simulink library "VisualAqSurveillanceBlock_devAlt"  (R2019b)
settings: Solver=VariableStepAuto  StartTime=0.0  StopTime=10.0  RelTol=1e-3
undefined symbols (not defined in the file): visaq_alert, visaq_area_s, visaq_beta0, visaq_beta1, visaq_d1, visaq_dlim, visaq_fovd, visaq_fovl, visaq_fovr, visaq_fovu, visaq_pl, visaq_pr, visaq_r, visaq_rseed, visaq_t1, visaq_t2, visaq_vdf, visaq_vis
libraries: CreateCovDiagMatrix x1, simulink x1
settings Model: Creator=BI28030  LastModifiedBy=ng21251
settings DataIOCC: ReturnWorkspaceOutputs=off
settings DebuggingCC: ArithmeticOperatorsInVariantConditions=warning
settings SFSimCC: CustomCodeUndefinedFunction=UseInterfaceOnly

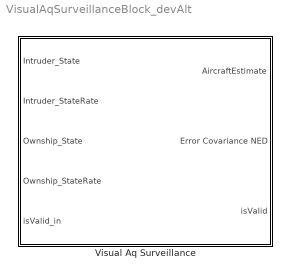
== system VisualAqSurveillanceBlock_devAlt ==
  Visual Aq Surveillance : Subsystem  Description=|  mask{dt=0.1, area_s=visaq_area_s, t2=visaq_t2, t1=visaq_t1, d1=visaq_d1, pl=visaq_pl, pr=visaq_pr, fovl=visaq_fovl, fovr=visaq_fovr, fovu=visaq_fovu, fovd=visaq_fovd, beta0=visaq_beta0, beta1=visaq_beta1, alert=visaq_alert, r=visaq_r, dlim=visaq_dlim, vis=visaq_vis, vdf=visaq_vdf, rseed=visaq_rseed}
      | Documentation for Perfect Observation Block                                                                                                                                                                                                                                                                                                                                                                                                          
      |                                                                                                                                                                                                                                                                                                                                                                                                                                                      
      | Description:  The perfect observation block, also known as a perfect                                                                                                                                                                                                                                                                                                                                                                                 
      | surveillance block, receives an Aircraft State, nominally from a Basic                                                                                                                                                                                                                                                                                                                                                                               
      | Aircraft Dynamics block, and outputs an Aircraft Estimate.  The Aircraft                                                                                                                                                                                                                                                                                                                                                                             
      | State that is received as input consists of Latitude, Longitude, and                                                                                                                                                                                                                                                                                                                                                                                 
      | Altitude state information as well as the aircraft position in local                                                                                                                                                                                                                                                                                                                                                                                 
      | coordinates in units of feet for north, east, and height.  The Aircraft                                                                                                                                                                                                                                                                                                                                                                              
      | Estimate outputs consist of estimates for the aircraft Latitude, Longitude, and Altitude, the east, north up position, and sensor covariance.  For perfect surveillance, the covariance estimates are all set to zero as default.  In addition, "time of validity" and a Boolean flag for the sensor report, "is Valid", are outputted as part of the Aircraft Estimate.                                                                             
      |                                                                                                                                                                                                                                                                                                                                                                                                                                                      
      | The initial perfect surveillance block developed receives the aircraft state information from the "AC2 - Basic Aircraft Dynamics" block within the "nominalEncounter" study.  Since the expected output from the AC1 and AC2 aircraft states have slightly different output parameters than what is provided from the perfect surveillance block (i.e., covariance estimates, isValid, and time of validity), the perfect surveillance block         
      | AircraftEstimate output has been left disconnected.                                                                                                                                                                                                                                                                                                                                                                                                  
      |                                                                                                                                                                                                                                                                                                                                                                                                                                                      
      | The initial unit test performed for this perfect observation block was to                                                                                                                                                                                                                                                                                                                                                                            
      | run the nominalEncounter study and to ensure that the simulation completes and no exceptions are encountered.  This unit test was successful (other than receiving a warning that the output of the perfect surveillance block is not connected, which was expected).  A more comprehensive future unit test would be to evaluate the position inputs and compare them with the position outputs to ensure that they are consistent with one another.
      mask prompts: dt "Dynamics Update Step Size (s)"; area_s "Aircraft Surface Area Array"; t2 "Evaluation Period (seconds)"; t1 "Alert Evaluation Period (seconds)"; d1 "Alert Evaluation Distance (nm)"; pl "Left Pilot Search Rate (0-1)"; pr "Right Pilot Search Rate (0-1)"; fovl "Pilot FOV Left (degrees ex:-110)"; fovr "Pilot FOV Right (degrees ex: 90)"; fovu "Pilot FOV Up (degrees ex:30)"; fovd "Pilot FOV Down (degrees ex: -20)"; beta0 "Beta for unalerted search (17000)"; beta1 "Beta for alerted search (14000)"; alert "Use Alerting Flag (1=yes, 0=no)"; r "R visual range (nm)"; dlim "Resolution limit of eye (arc-min)"; vis "visbility factor (0-1)"; vdf "visual degredation factor (0-1)"; rseed "Random seed for uniform distribution (0-1)"

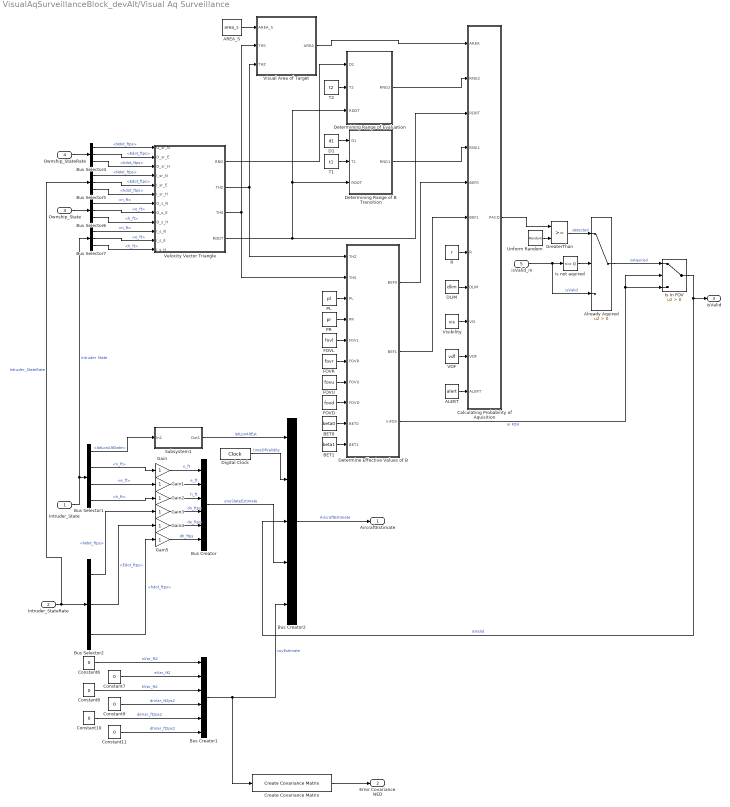
== system VisualAqSurveillanceBlock_devAlt/Visual Aq Surveillance ==
  Intruder_State : Inport  OutDataTypeStr=Bus: AircraftState
  Intruder_StateRate : Inport  Port=2  OutDataTypeStr=Bus: AircraftStateRate
  Ownship_State : Inport  Port=3  OutDataTypeStr=Bus: AircraftState
  Ownship_StateRate : Inport  Port=4  OutDataTypeStr=Bus: AircraftStateRate
  isValid_in : Inport  Port=5
  ALERT : Constant  Value=alert
  "AREA_S " : Constant  Value=area_s  VectorParams1D=off
  Already Aquired : Switch  Criteria=u2 > Threshold
  BET0 : Constant  Value=beta0
  BET1 : Constant  Value=beta1
  Bus Creator : BusCreator  Inputs=6  OutDataTypeStr=Bus: StateEstimate
  Bus Creator1 : BusCreator  Inputs=6  OutDataTypeStr=Bus: CovarianceEstimate
  Bus Creator2 : BusCreator  Inputs=5  OutDataTypeStr=Bus: AircraftEstimate  NonVirtualBus=on
  Bus Selector1 : BusSelector  OutputSignals=latLonAltState,n_ft,e_ft,h_ft
  Bus Selector2 : BusSelector  OutputSignals=Ndot_ftps,Edot_ftps,hdot_ftps
  Bus Selector4 : BusSelector  OutputSignals=Ndot_ftps,Edot_ftps,hdot_ftps
  Bus Selector5 : BusSelector  OutputSignals=Ndot_ftps,Edot_ftps,hdot_ftps
  Bus Selector6 : BusSelector  OutputSignals=n_ft,e_ft,h_ft
  Bus Selector7 : BusSelector  OutputSignals=n_ft,e_ft,h_ft
  Calculating Probability of Aquisition : MATLAB Function  TreatAsAtomicUnit=on
  Constant{6..11} (6 alike) : Constant  Value=0
  Create Covariance Matrix : CreateCovDiagMatrix/Create Covariance Matrix  SystemSampleTime=-1  Latency=0  AutoFrameSizeCalculation=off
  D1 : Constant  Value=d1
  DLIM : Constant  Value=dlim
  Determine Effective Values of B : MATLAB Function  TreatAsAtomicUnit=on
  Determining Range of B Transition : MATLAB Function  TreatAsAtomicUnit=on
  Determining Range of Evaluation : MATLAB Function  TreatAsAtomicUnit=on
  Digital Clock : DigitalClock  SampleTime=dt
  FOVD : Constant  Value=fovd
  FOVL : Constant  Value=fovl
  FOVR : Constant  Value=fovr
  FOVU : Constant  Value=fovu
  Gain{,1..5} (6 alike) : Gain
  GreaterThan : RelationalOperator  OutDataTypeStr=boolean  RndMeth=Simplest
  Is In FOV : Switch  Criteria=u2 > Threshold
  PL : Constant  Value=pl
  PR : Constant  Value=pr
  R : Constant  Value=r
  Subsystem1 : Subsystem
  T1 : Constant  Value=t1
  T2 : Constant  Value=t2
  Unform Random : UniformRandomNumber  Minimum=0  Seed=rseed  SampleTime=0.1
  VDF : Constant  Value=vdf
  Velocity Vector Triangle : MATLAB Function  TreatAsAtomicUnit=on
  Visibility : Constant  Value=vis
  Visual Area of Target : MATLAB Function  TreatAsAtomicUnit=on
  is not aquired : simulink/Logic and Bit Operations/Compare To Zero  relop=<=  OutDataTypeStr=boolean
  AircraftEstimate : Outport  OutDataTypeStr=Bus: AircraftEstimate  VectorParamsAs1DForOutWhenUnconnected=off
  Error Covariance NED : Outport  Port=2  VectorParamsAs1DForOutWhenUnconnected=off
  "isValid " : Outport  Port=3
  wires:
  Gain5/1 -> Bus Creator/6  "dh_ftps"
  Gain4/1 -> Bus Creator/5  "de_ftps"
  Gain3/1 -> Bus Creator/4  "dn_ftps"
  Gain2/1 -> Bus Creator/3  "h_ft"
  Gain1/1 -> Bus Creator/2  "e_ft"
  Gain/1 -> Bus Creator/1  "n_ft"
  Subsystem1/1(Out1) -> Bus Creator2/1  "latLonAltEst"
  Digital Clock/1 -> Bus Creator2/2  "timeOfValidity"
  isValid_in/1 -> is not aquired/1, Already Aquired/3  "isValid"
  Bus Selector1/1 -> Subsystem1/1(In1)  "<latLonAltState>"
  Bus Selector2/3 -> Gain5/1  "<hdot_ftps>"
  Bus Selector2/2 -> Gain4/1  "<Edot_ftps>"
  Bus Selector2/1 -> Gain3/1  "<Ndot_ftps>"
  Bus Selector1/4 -> Gain2/1  "<h_ft>"
  Bus Selector1/3 -> Gain1/1  "<e_ft>"
  Bus Selector1/2 -> Gain/1  "<n_ft>"
  Constant11/1 -> Bus Creator1/6  "dhVar_ft2ps2"
  Constant10/1 -> Bus Creator1/5  "deVar_ft2ps2"
  Constant9/1 -> Bus Creator1/4  "dnVar_ft2ps2"
  Constant8/1 -> Bus Creator1/3  "hVar_ft2"
  Constant7/1 -> Bus Creator1/2  "eVar_ft2"
  Constant6/1 -> Bus Creator1/1  "nVar_ft2"
  Bus Creator2/1 -> AircraftEstimate/1  "AircraftEstimate"
  Bus Creator1/1 -> Create Covariance Matrix/1, Bus Creator2/5  "covEstimate"
  Bus Creator/1 -> Bus Creator2/4  "enuStateEstimate"
  Create Covariance Matrix/1 -> Error Covariance NED/1
  Intruder_State/1 -> Bus Selector7/1, Bus Selector1/1  "Intruder State"
  Intruder_StateRate/1 -> Bus Selector5/1, Bus Selector2/1  "Intruder_StateRate"
  Bus Selector4/3 -> Velocity Vector Triangle/3(O_sr_H)  "<hdot_ftps>"
  Bus Selector4/1 -> Velocity Vector Triangle/1(O_sr_N)  "<Ndot_ftps>"
  Bus Selector4/2 -> Velocity Vector Triangle/2(O_sr_E)  "<Edot_ftps>"
  Ownship_StateRate/1 -> Bus Selector4/1
  Bus Selector5/2 -> Velocity Vector Triangle/5(I_sr_E)  "<Edot_ftps>"
  Bus Selector5/3 -> Velocity Vector Triangle/6(I_sr_H)  "<hdot_ftps>"
  Bus Selector5/1 -> Velocity Vector Triangle/4(I_sr_N)  "<Ndot_ftps>"
  Ownship_State/1 -> Bus Selector6/1
  Bus Selector6/3 -> Velocity Vector Triangle/9(O_s_H)  "<h_ft>"
  Bus Selector6/1 -> Velocity Vector Triangle/7(O_s_N)  "<n_ft>"
  Bus Selector6/2 -> Velocity Vector Triangle/8(O_s_E)  "<e_ft>"
  Bus Selector7/3 -> Velocity Vector Triangle/12(I_s_H)  "<h_ft>"
  Bus Selector7/1 -> Velocity Vector Triangle/10(I_s_N)  "<n_ft>"
  Bus Selector7/2 -> Velocity Vector Triangle/11(I_s_E)  "<e_ft>"
  Velocity Vector Triangle/4(RDOT) -> Calculating Probability of Aquisition/3(RDOT), Determining Range of Evaluation/3(RDOT), Determining Range of B Transition/3(RDOT)
  Velocity Vector Triangle/3(THS) -> Determine Effective Values of B/2(THS), Visual Area of Target/2(THS)
  D1/1 -> Determining Range of B Transition/1(D1)
  T1/1 -> Determining Range of B Transition/2(T1)
  T2/1 -> Determining Range of Evaluation/2(T2)
  Velocity Vector Triangle/1(RNG) -> Determining Range of Evaluation/1(D2)
  PL/1 -> Determine Effective Values of B/3(PL)
  PR/1 -> Determine Effective Values of B/4(PR)
  FOVL/1 -> Determine Effective Values of B/5(FOVL)
  FOVR/1 -> Determine Effective Values of B/6(FOVR)
  BET0/1 -> Determine Effective Values of B/9(BET0)
  BET1/1 -> Determine Effective Values of B/10(BET1)
  Determining Range of B Transition/1(RNG1) -> Calculating Probability of Aquisition/4(RNG1)
  Visual Area of Target/1(AREA) -> Calculating Probability of Aquisition/1(AREA)
  Determining Range of Evaluation/1(RNG2) -> Calculating Probability of Aquisition/2(RNG2)
  Determine Effective Values of B/1(BEF0) -> Calculating Probability of Aquisition/5(BEF0)
  Determine Effective Values of B/2(BEF1) -> Calculating Probability of Aquisition/6(BEF1)
  DLIM/1 -> Calculating Probability of Aquisition/8(DLIM)
  R/1 -> Calculating Probability of Aquisition/7(R)
  Velocity Vector Triangle/2(THZ) -> Determine Effective Values of B/1(THZ), Visual Area of Target/3(THZ)
  FOVU/1 -> Determine Effective Values of B/7(FOVU)
  FOVD/1 -> Determine Effective Values of B/8(FOVD)
  Calculating Probability of Aquisition/1(PACQ) -> GreaterThan/1
  Unform Random/1 -> GreaterThan/2
  GreaterThan/1 -> Already Aquired/1  "detected"
  is not aquired/1 -> Already Aquired/2
  Determine Effective Values of B/3(inFOV) -> Is In FOV/3, Is In FOV/2  "in FOV"
  Already Aquired/1 -> Is In FOV/1  "isAquired"
  Is In FOV/1 -> "isValid "/1, Bus Creator2/3  "isValid"
  VDF/1 -> Calculating Probability of Aquisition/10(VDF)
  Visibility/1 -> Calculating Probability of Aquisition/9(VIS)
  "AREA_S "/1 -> Visual Area of Target/1(AREA_S)
  ALERT/1 -> Calculating Probability of Aquisition/11(ALERT)

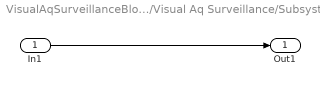
== system VisualAqSurveillanceBlock_devAlt/Visual Aq Surveillance/Subsystem1 ==
  In1 : Inport
  Out1 : Outport  VectorParamsAs1DForOutWhenUnconnected=off
  wires:
  In1/1 -> Out1/1

== matlab function VisualAqSurveillanceBlock_devAlt/Visual Aq Surveillance/Velocity Vector Triangle ==
  data: RNG output; THZ output; O_sr_N input; THS output; O_sr_E input; RDOT output; O_sr_H input; I_sr_N input; I_sr_E input; I_sr_H input; O_s_N input; O_s_E input; O_s_H input; I_s_N input; I_s_E input; I_s_H input
function [RNG, THZ, THS, RDOT] = JAndrews_Mod_2(O_sr_N,O_sr_E,O_sr_H,I_sr_N,I_sr_E,I_sr_H,O_s_N,O_s_E,O_s_H,I_s_N,I_s_E,I_s_H)
% Input variable defintions
% No, symbol, name, value, definition
% 1.  - , BET0, 17000 per steradian-sec,  single pilot B values before transition
% 2.  - , BET1, 17000 per steradian-sec,  Single-pilot B value after transition
% 3.  t1, T1,   180 sec,                  modified tau time for B transition (time to closest approach)
% 4.  t2, T2,   12 sec,                   modified tau time for evaluation of PACQ (time to closest approach)
% 5.  D1, D1,   0. nmi,                   modified tau range parameter for B transition.
% 6.  D2, D2,   0. nmi,                   modified tau range parameter for PACQ evaluation
% 7.  R,  R,    20. nmi,                  visual range
% 8.  d,  DLIM, 1 arc-min,                Resolution limit of human eye.
% 9.  V1, VSUB1,180 kt,                   airspeed of subject aircraft.
% 10. V2, VSUB2,130 kt,                   airspeed of target aircraft.
% 11. - , IACT, 1,                        aircraft type for target aircraft (see table)
% 12. X,  XANG, 180. deg,                 Crossing angle (relative heading)
% 13. PL, PL,   1.0,                      Search intensity for pilot in left seat (0 = no pilot, 1 = normal search)
% 14. PR, PR,   1.0,                      Search intensity for pilot in right seat (0 = no pilot, 1 = normal search)
% 15. FL, FOVL, -120 degrees              Field-of-view cutoff on left side for searching pilot in left seat (measured positive clockwise from straight ahead). 
% 16. FR, FOVR, -90 degrees               Field-of-view cutoff on left side for searching pilot in right seat (measured positive clockwise from straight ahead). 
% 17. r., RDOT, 380 kt*,                  Range rate of target aircraft
% 18. Ax, AX,   35 sq.ft.*,               Head-on visual area of target.
% 19. Ay, AY,   85 sq.ft.*,               Broadside visual area of target.
% 20. Az, AZ,   260 sq.ft.*,              Topside visual area of target.
% 21. A,  AREA, 35 sq.ft.*,               Final visual area of target.
% 22. 0T, TH1(THS),  0 deg*,                   Bearing of target aircraft as seen from subject aircraft.
% 23. 0S, TH2(THT),  0 deg*,                   Bearing of subject aircraft as seen from target aircraft.
% 24. R1, RNG1, 3.78 nmi*,                Range at which B transition occurs.
% 25. R2, RNG2, 1.27 nmi*,                Range at which PACQ is evaluated.
% 26. B0, BEF0, 17000* per steradian-sec, Effective value of B before transition.
% 27. B1, BEF1, 17000* per steradian-sec, Effective value of B after transition.
% 28. P, PACQ,  -                         Probability of visual aquisition
% *=value that is computed when all 16 input variables have nominal value.

%% Module 2 Description - - - - - - - 
% From a knowledge of the aircraft airspeeds and the croesing angle,
% Module 2 solves the velocity vector triangle (Fig. 4.4) to determine the
% epPrOach bearings and range rate. This solution assumes that the aircraft are
% on a rectilinear collision course and hence that the horizontal fiss distance
% is zero. For theee conditions, the valuea of the range rate (R~) and the
% approach bearings (THS and THT) are constant.

% Approach bearings are meaeured positive clockwise from straight ahead and
% are expreesed as a number between -180 degraes and +180 degreee. me crossing
% angle, NG, ie simply the relative heading formed by subtracting the headiog
% of the target aircraft from the heading of the subject aircraft. The simple
% trigonometric formula that relatee the approach bearinge and the crossing
% angle is

% WG = 180° + THS - THT

% me approach bearing for the target aircraft (THT) is important since it
% detetines the vieual area that will be seen from the subject aircraft (see
% discussion in 4.2.3). The approach bearing for the subject (~S) is usad in
% Module 4 to determine whethar or not the target ia within the cockpit
% field-of~few.

%% --------------------Module 2 ------------------
%Output
%THT - 
%THS (degrees)
%RDOT (knots)
%RNG (nm)

%get heading of Ownship (degrees)
VSUB=rad2deg(pi/2 - atan2(O_sr_N, O_sr_E));

%get heading of intruder (degrees)
VTAR=rad2deg(pi/2 - atan2(I_sr_N, I_sr_E));

%bearing to intruder (from ownship) (degrees)

    %intruder location (if ownship was at 0,0)
    Int_loc=[I_s_N - O_s_N, I_s_E - O_s_E];

    %Bearing to intruder from ownship (degrees)
    THS = rad2deg( pi/2 - atan2( Int_loc(1), Int_loc(2) ) );
    
%bearing to ownship (from intruder) (degrees)

    %ownship location (if intruder was at 0,0)
    Own_loc=[O_s_N - I_s_N, O_s_E - I_s_E];
    
    %bearing to ownship from intruder (degrees)
    THT = rad2deg( pi/2 - atan2( Own_loc(1), Own_loc(2) ) );

%check that intruder & own bearings math is correct.
% assert(isequal(ceil(sum(THT,THS)),360));

%calculate the difference between headings
XANG= 180 + THS - THT;

%Calculate RDOT - range rate
RDOT_ftsec = ( (I_sr_N - O_sr_N)^2 + (I_sr_E - O_sr_E)^2 )^(1/2);
RDOT = RDOT_ftsec * 60*60 / 6076.115486; %now in knots

%Calculate THZ in degrees

    %calculate adjacent - horizontal distance
    H_dist = ( (I_s_N - O_s_N)^2 + (I_s_E - O_s_E)^2 )^0.5;

    %calculate opposite - vertical distance
    V_dist = I_s_H - O_s_H;

    %calculate vertical angle
    THZ = rad2deg( atan(V_dist / H_dist));
    
RNG = ( (I_s_N - O_s_N)^2 + (I_s_E - O_s_E)^2 )^(1/2);

== matlab function VisualAqSurveillanceBlock_devAlt/Visual Aq Surveillance/Visual Area of Target ==
  data: AREA_S input; AREA output; THS input; THZ input
function AREA = JAndrews_Mod_3(AREA_S, THS, THZ)
% Input variable defintions
% No, symbol, name, value, definition
% 18. Ax, AX,   35 sq.ft.*,               Head-on visual area of target.
% 19. Ay, AY,   85 sq.ft.*,               Broadside visual area of target.
% 20. Az, AZ,   260 sq.ft.*,              Topside visual area of target.
% 21. A,  AREA, 35 sq.ft.*,               Final visual area of target.
% 22. 0T, TH1,  0 deg*,                   Bearing of target aircraft as seen from subject aircraft.
% 23. 0S, TH2,  0 deg*,                   Bearing of subject aircraft as seen from target aircraft.
% 24. R1, RNG1, 3.78 nmi*,                Range at which B transition occurs.
% 25. R2, RNG2, 1.27 nmi*,                Range at which PACQ is evaluated.
% 26. B0, BEF0, 17000* per steradian-sec, Effective value of B before transition.
% 27. B1, BEF1, 17000* per steradian-sec, Effective value of B after transition.
% 28. P, PACQ,  -                         Probability of visual aquisition
% *=value that is computed when all 16 input variables have nominal value.



%%-------MODULE 3---------
% 4.2.3 Module 3: Computing the Visual Area of the Target
% The visual area of the target ie computed by projecting the principal
% visual areas AX and AY onto a plane that is normal to the linemf-sfght
% between the two aircraft. ~is plane is at an angle ~ with respect to the
% Y-Z plane for the target aircraft. h approximate correction for shielding ie
% applied by assudng that the actual visual area is the largest of the
% projectione of M and AY plus one+hird of the smallest projection (see
% Mference 2). ~is approximation is errorless when the aircraft ie viewed
% along one of the principal axas. Because Mdule 3 assumes that the
% line-f =ight lies tithin the X-Y plane, the topside area, AZ, ie not allowed
% to centribute to the target visual area. This ia normally a good assumption,
% but can result in underestimation of the visual area if the pitch angle of the
% aircraft is large. U is defined in the module to allow for future exteneion
% of the software.




    
    THSdiff=abs(AREA_S(:,1)-THS);
    THZdiff=abs(AREA_S(:,2)-THZ);
    TOTdiff=THSdiff+THZdiff;
    mindiff=min(TOTdiff);
    
    %find the closest angle combination
    indx=ismember(TOTdiff,mindiff);
    
    %make a list of indicies
    %find the incidices that are the closest
    %take the first instance only
    indxnum=1:numel(indx);
    indxnum=indxnum(indx>0);
    indxnum=indxnum(1);
    
    %area = first smallest index - convert to nm^2
    AREA=AREA_S(indxnum,3)/6076.115486;
    
    
% else
% 
% XArea = abs(cos(deg2rad(THS))) * abs(cos(deg2rad(THZ))) * AX;
% YArea = abs(sin(deg2rad(THS))) * abs(cos(deg2rad(THZ))) * AY;
% 
% ZArea = abs(sin(deg2rad(THZ))) * AZ;
% 
% 
% 
% AREA = XArea + YArea + ZArea;
% AREA=AREA/6076.115486;
% end

== matlab function VisualAqSurveillanceBlock_devAlt/Visual Aq Surveillance/Determining Range of B Transition ==
  data: D1 input; RNG1 output; T1 input; RDOT input
function RNG1 = JAndrews_Mod_6(D1,T1,RDOT)
% Input variable defintions
% No, symbol, name, value, definition
% 3.  t1, T1,   180 sec,                  modified tau time for B transition (time to closest approach)
% 5.  D1, D1,   0. nmi,                   modified tau range parameter for B transition.
% 17. r., RDOT, 380 kt*,                  Range rate of target aircraft
% 24. R1, RNG1, 3.78 nmi*,                Range at which B transition occurs.
% *=value that is computed when all 16 input variables have nominal value.

%% Modeule 6 -
% 4.2.6 Wdule 6: Determining the tinge of 8 Transition
% In a particular scenario, the nominal value of 6 for a single pilot mey
% be alterad by an event such as the receipt of a traffic advieory.SEE1 allowa
% the notinal single~ilot value of 6 to transition from one value to another at
% a predefined point during the encounter. The initial value of 6 is BETO.
% After the transition, the value of B fa BET1 (see Fig. 4.6). The range at
% which trzaaition occurs ia NG1. It is computed using a modified tau
% criterion involving the two input parameter DI and RI:
% 
% RNG1 = D1 - ROOT*T1
% 
% The transition occurs when the target is T1 secondefrom reaching a
% range D1. Note that if TI=O, then a simple range criterion results. H D1=O,
% then a simple time-to-collision criterion reeulta.
% If the application of interest does not require a transition, the
% transition ie easily avoided by setting BET1 equal to BETO. The eettings of
% D1 and T1 then have no effect upon the computations (becauae the valuee of 8
% are unchanged by reaching the transition point).

%RNG1 = D1 (0 nmi) - RDOT (kts) * T1 (seconds)

RNG1 = D1 - RDOT * T1;

== matlab function VisualAqSurveillanceBlock_devAlt/Visual Aq Surveillance/Determining Range of Evaluation ==
  data: D2 input; RNG2 output; T2 input; RDOT input
function RNG2 = JAndrews_Mod_5(D2, T2, RDOT)
% Input variable defintions
% No, symbol, name, value, definition
% 4.  t2, T2,   12 sec,                   modified tau time for evaluation of PACQ (time to closest approach)
% 6.  D2, D2,   0. nmi,                   modified tau range parameter for PACQ evaluation
% 17. r., RDOT, 380 kt*,                  Range rate of target aircraft
% 25. R2, RNG2, 1.27 nmi*,                Range at which PACQ is evaluated.
% *=value that is computed when all 16 input variables have nominal value.

%%  4.2.5 Module 5: Determining the ~nge of Evaluation
% The cumulative probability of visual acquisition, PACQ, depends upon the
% range, MG2, at which PACQ ia to be evaluated: Often it ia desirable to aet
% this ranga to the latest point at which sufficient time exists for evasive
% action. Then PACQ till repreeent tha probability of visual acquisition with
% aufficient lead time for avoidanca.
% RNG2 ie computed using a modified tau criterion based upon two input
% parameter D2 and U:
% ~G2 = D2 - ~OT*T2
% From thie equation it can be seen that SNG2 ie reached when tbe target
% ia T2 seconds from reaching a range of D2. with this formulation, WG2 can
% be deterdned as either a constant range, a constant time-to-collision, or a
% modified tau criterion. For example, if T2=0, then the equation yields a
% simple range critaria for which PACQ is evaluated at range D2. If D2=0,
% then a simple time critaria results in which PACQ La evaluated when T2
% secoada remain befora collision. If neither T2 nor D2 are zero, then a
% modified tau criterion results.

%RNG2 = D2 (0 nmi) - RDOT (kts) * T2 (12 seconds)

RNG2 = D2 - RDOT * T2;

== matlab function VisualAqSurveillanceBlock_devAlt/Visual Aq Surveillance/Determine Effective Values of B ==
  data: THZ input; THS input; BEF0 output; PL input; PR input; FOVL input; FOVR input; FOVU input; FOVD input; BET0 input; BET1 input; BEF1 output; inFOV output
function [BEF0, BEF1,inFOV] = JAndrews_Mod_4(THZ, THS, PL, PR, FOVL, FOVR, FOVU, FOVD, BET0, BET1)
% Input variable defintions
% No, symbol, name, value, definition
% 1.  - , BET0, 17000 per steradian-sec,  single pilot B values before transition
% 2.  - , BET1, 17000 per steradian-sec,  Single-pilot B value after transition
% 13. PL, PL,   1.0,                      Search intensity for pilot in left seat (0 = no pilot, 1 = normal search)
% 14. PR, PR,   1.0,                      Search intensity for pilot in right seat (0 = no pilot, 1 = normal search)
% 15. FL, FOVL, -120 degrees              Field-of-view cutoff on left side for searching pilot in left seat (measured positive clockwise from straight ahead). 
% 16. FR, FOVR, 90 degrees               Field-of-view cutoff on left side for searching pilot in right seat (measured positive clockwise from straight ahead). 
% 23. 0S, TH2(THT),  0 deg*,              Bearing of subject aircraft as seen from target aircraft.
% 26. B0, BEF0, 17000* per steradian-sec, Effective value of B before transition.
% 27. B1, BEF1, 17000* per steradian-sec, Effective value of B after transition.
% 28. P, PACQ,  -                         Probability of visual aquisition
% *=value that is computed when all 16 input variables have nominal value.

%% 4.2.4 Module 4: Wtermining the Effective Values of 6
% Module 4 examinee cockpit visibility and crew complement in order to
% deterfine their effect upon search effectiveness. It does eo by taking the
% notinal single~ilot B values and ebng them to produce effective B
% values. For a single pilot devoting normal effort to visual search, the
% value of S before and afterthetransitionevent(eee4.2.6)are represented
% by parameter BETO and BET1. Module 4 computes two corresponding effective
% 8 values, BEFO and BEF1, by e-rig the 8 values for each pilot who ie able to
% contribute to visual search.
% 
% The fieldmf~iew of the cockpit is deter~ned by the variables FOW and
% FOPS (ace Fig. 4.5). It ia aesumed that the cockpit visibility ia symmetric
% and that there is no cut~ff in elevation (normally true for targeta on
% collision courses). Tfienthe target ~a outside the field-f -iew, the
% effective 6 velue is set to zero.
% By setting FL and ~, the user specifies the number of pilots that
% contribute to search for both left and right visibility limite. Normally PL
% and ~ are efther sero (no pilot in the seat) or unity (single pilot in seat
% and eearching normally). It is possible to use a value between O and 1 to
% represent a pilot who is preeent, but ia devoting less than the normal amount
% of time to visual search. Or a value greater than 1 can be used to represent
% search by an additional crew member.
% 
% For the nominal input values given in Table 3.1, it ia assumed that a
% single pilot is searching from the left seat of the aircraft (PL=l.O, pR=O.O).
% For the notinal values of croesing angle (WG-180 degrees), tha intruder is
% always within the field of view. Thus for the nominal input values, BEFO=BETO
% and BEF1=BET1.

%% CHECK FOR FOV L/R PILOT

%THS is now between -180 and 180;
while THS<-180
    THS=THS+360;
end
while THS>180
    THS=THS-360;
end
    
%ensure THZ is between +/-90
if THZ>360
    THZ=mod(THZ,360);
end
if THZ>90
    THZ=THZ-360;
end
 

% if left pilot present
PL_FOV = 0;
if PL
    
    %check if intruder w/in field of view
    if THS >= FOVL && THS <= FOVR &&...  %target is w/in L/R LOS
            ( (THZ >= FOVD && THZ <= FOVU) ||... %THZ is -90 to +90
            (THZ > FOVU && THZ >= FOVD + 360 && THZ < 360) ) %THZ is >270
        
            PL_FOV = 1;
        
    end
else
    PL_FOV = 0;
end

%check if right pilot present
PR_FOV=0;
if PR 
        if THS >= -FOVR && THS <= -FOVL &&...  %target is w/in L/R LOS
            ( (THZ >= FOVD && THZ <= FOVU) ||... %THZ is -90 to +90
            (THZ > FOVU && THZ >= FOVD + 360 && THZ < 360) ) %THZ is >270
        
            PR_FOV = 1;
        end
else
    PR_FOV=0;
end
        
        
%set BETs = BEFs
BEF0 = BET0 * PL_FOV + BET0 * PR_FOV;
BEF1 = BET1 * PL_FOV + BET1 * PR_FOV;

inFOV=PL_FOV||PR_FOV;

== matlab function VisualAqSurveillanceBlock_devAlt/Visual Aq Surveillance/Calculating Probability of Aquisition ==
  data: AREA input; PACQ output; RNG2 input; RDOT input; RNG1 input; BEF0 input; BEF1 input; R input; DLIM input; VIS input; VDF input; ALERT input
function PACQ = JAndrews_Mod_7(AREA, RNG2, RDOT, RNG1, BEF0, BEF1, R, DLIM, VIS, VDF,ALERT)
% Input variable defintions
% No, symbol, name, value, definition
% 7.  R,  R,    20. nmi,                  visual range
% 8.  d,  DLIM, 1 arc-min,                Resolution limit of human eye.
% 17. r., RDOT, 380 kt*,                  Range rate of target aircraft
% 21. A,  AREA, 35 sq.ft.*,               Final visual area of target.
% 24. R1, RNG1, 3.78 nmi*,                Range at which B transition occurs.
% 25. R2, RNG2, 1.27 nmi*,                Range at which PACQ is evaluated.
% 26. B0, BEF0, 17000* per steradian-sec, Effective value of B before transition.
% 27. B1, BEF1, 17000* per steradian-sec, Effective value of B after transition.
% 28. P, PACQ,  -                         Probability of visual aquisition
% *=value that is computed when all 16 input variables have nominal value.
 
%ALERT a new variable which enables alerting or not for the run.
 
% 4.2.7 Module 7: timputing the Wmulative Probability of kquiaition
% M
% Module 7 ia the final module that actually computes the probability of
% visual acquisition, PACQ. It requires 8 inputa aa ahom in Fig. 4.1.
% Module 7 aaaumes that the acquisition rate drops immediately to zero when
% the target ia beyond a range, RLIM, corresponding to the resolution limit of
% the human eye. RLIM ia defined aa follows: First, DL~, WA, and RDOT are
% used to compute the range at which the solid angle subtended by the target
% equals that of a circle with diameter DL~. This range ia given by the
% formula
% 1.1284*SQRT(AREA)/DLIM
% where DL~ ia in radiana. Then, if this range is greater than R, the visual
% range, it is reduced to R. The net result ia
% RLIM = ndnimum [1.1284*SQRT(A~A)/DLIM, R]
% A more aophieticated model for MIM could be constructed, but in meet
% analyaea, only a tiny fraction of the opportunity for visual acquieition
% occurs before the target ie well within visual range and well above the
% resolution threshold. Wnce, the detaile of the model in this regard are
% normally of little consequence.
% Note that if RLIM ia less than RNGl, then % till already have
% transitioned to BET1 before the target is close enough to be seen. b this
% caae, the value of BETO has no affect upon the calculation.
 
%Range limit = the minimum of either the human eye distinguishing target size or visual range
RLIM = min([ 1.1284 * (AREA)^0.5 / DLIM, R]);

%if the eval range is beyond these two - cannot detect
if RNG2 > RLIM 
    PACQ=0;
    
else
    
%else
    rng3=intcalcforce(AREA,RNG2,RDOT);
    pacq_3= BEF0*(rng3)*VIS*VDF;
    PACQ=1.0-exp(-pacq_3);

end


function x_e = intcalcforce(A,B,C)
T2=0:0.0001:0.1;

tmp=(A./(B+C*T2).^2).* exp(-2.996 * (B+C*T2));
x_e=sum(tmp*0.0001)*((numel(T2)-1)/numel(T2));
